simulink model "regen"  (R2025b)
settings: Solver=FixedStepAuto  StartTime=0.0  StopTime=55  FixedStep=0.005  RelTol=1e-3
InitFcn:
  | speed_min = 6;
  | bpt_fmax = 60;
  | bpt_rmax = 60;
  | voltage_max = 299;
  | pedals_max = 0;
model workspace (MAT data in the model file):
  efficiency_grid = [0  0  0  0  0  0  0  0  0  0  0; 0  0.86  0.88  0.89  0.89  0.89  0.89  0.88  0.86  0.8  0.8; 0  0.88  0.94  0.94  0.95  0.95  0.94  0.94  0.94  0.88  0.85; 0  0.88  0.94  0.95  0.96  0.96  0.96  0.96  0.95  0.94  0.86; 0  0.88  0.94  0.95  0.96  0.95  0.95  0.95  0.95  0.94  0.93; 0  0.86  0.91  0.94  0.94  0.94  0.94  0.94  0.94  0.94  0.94; 0  0.83  0.88  0.92  0.92  0.92  0.92  0.92  0.92  0.91  0.9; 0  0.8  0.86  0.86  0.86  0.86  0.86  0.86  0.86  0.86  0.86]
  rpm_grid = [0  500  1000  1500  2000  2500  3000  3500  4000  4500  5000; 0  500  1000  1500  2000  2500  3000  3500  4000  4500  5000; 0  500  1000  1500  2000  2500  3000  3500  4000  4500  5000; 0  500  1000  1500  2000  2500  3000  3500  4000  4500  5000; 0  500  1000  1500  2000  2500  3000  3500  4000  4500  5000; 0  500  1000  1500  2000  2500  3000  3500  4000  4500  5000; 0  500  1000  1500  2000  2500  3000  3500  4000  4500  5000; 0  500  1000  1500  2000  2500  3000  3500  4000  4500  5000]
  torque_grid = [0  0  0  0  0  0  0  0  0  0  0; 20  20  20  20  20  20  20  20  20  20  20; 40  40  40  40  40  40  40  40  40  40  40; 60  60  60  60  60  60  60  60  60  60  60; 80  80  80  80  80  80  80  80  80  80  80; 100  100  100  100  100  100  100  100  100  100  100; 120  120  120  120  120  120  120  120  120  120  120; 140  140  140  140  140  140  140  140  140  140  140]
undefined symbols (not defined in the file or in its folder): DiscIntNeverNeededParam
libraries: simulink x4, sdolib x2
settings Model: Creator=benjaminlevin  LastModifiedBy=benjaminlevin

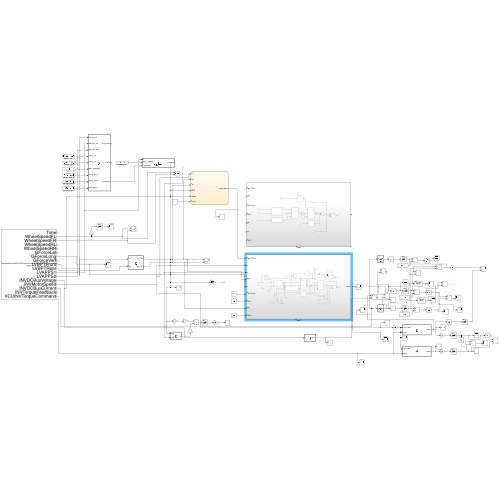
[thumbnail: Simulink's stored preview of the top-level diagram]
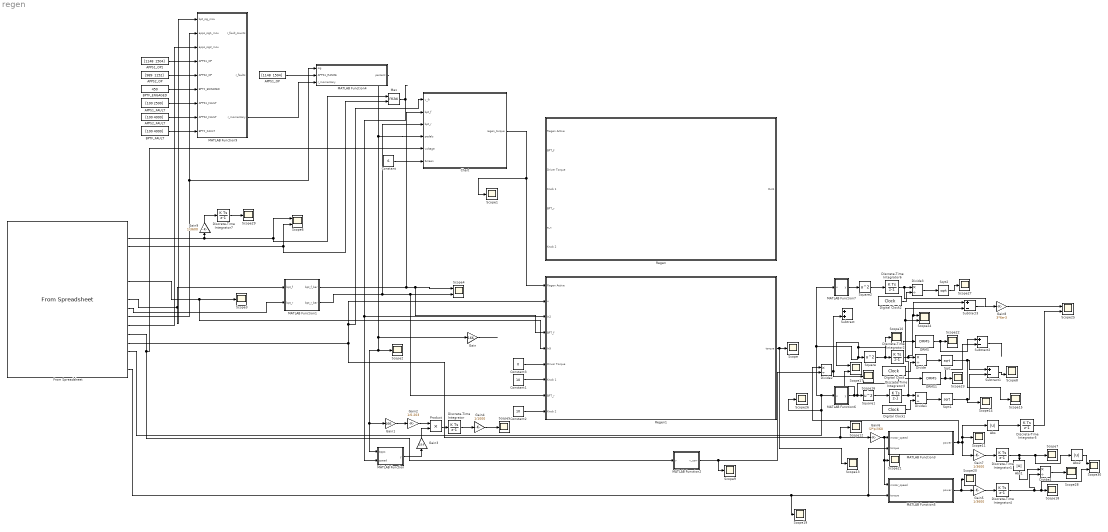
== system regen ==
  APPS1_FAULT : Constant  Value=[100 2500]  VectorParams1D=off
  APPS1_OP : Constant  Value="[1148  1504]"  VectorParams1D=off
  APPS1_OP1 : Constant  Value="[1148  1504]"  VectorParams1D=off
  APPS2_FAULT : Constant  Value=[100 4000]  VectorParams1D=off
  APPS2_OP : Constant  Value="[989  1152]"  VectorParams1D=off
  Abs : Abs  SaturateOnIntegerOverflow=off
  Abs1 : Abs  SaturateOnIntegerOverflow=off
  Abs2 : Abs  SaturateOnIntegerOverflow=off
  BPTF_ENGAGED : Constant  Value=450  VectorParams1D=off
  BPTF_FAULT : Constant  Value=[100 4000]  VectorParams1D=off
  Chart : Stateflow chart  TreatAsAtomicUnit=on
  Constant : Constant  Value=6
  Constant1 : Constant  Value=10
  Constant2 : Constant  Value=10
  Constant3 : Constant  Value=0
  DRMS : sdolib/RMS Blocks/DRMS  Ts=0.005
  DRMS1 : sdolib/RMS Blocks/DRMS  Ts=0.005
  Digital Clock : DigitalClock  SampleTime=0.005
  Digital Clock1 : DigitalClock  SampleTime=0.005
  Digital Clock2 : DigitalClock  SampleTime=0.005
  Discrete-Time Integrator{,1,4..5,7} (5 alike) : DiscreteIntegrator  SampleTime=-1  ICPrevOutput=DiscIntNeverNeededParam  ICPrevScaledInput=DiscIntNeverNeededParam
  Discrete-Time Integrator2 : DiscreteIntegrator  SampleTime=-1  SaturateOnIntegerOverflow=on  ICPrevOutput=DiscIntNeverNeededParam  ICPrevScaledInput=DiscIntNeverNeededParam
  Discrete-Time Integrator3 : DiscreteIntegrator  SampleTime=-1  SaturateOnIntegerOverflow=on  ICPrevOutput=DiscIntNeverNeededParam  ICPrevScaledInput=DiscIntNeverNeededParam
  Discrete-Time Integrator6 : DiscreteIntegrator  SampleTime=-1  SaturateOnIntegerOverflow=on  ICPrevOutput=DiscIntNeverNeededParam  ICPrevScaledInput=DiscIntNeverNeededParam
  Divide{,1..4} (5 alike) : Product  Inputs=*/
  From Spreadsheet : FromSpreadsheet  FileName=/Users/benjaminlevin/MATLAB/Projects/FormulaSAE/Simulations/regen_test2.xlsx  TreatFirstColumnAs=Data  SampleTime=0.005
  Gain : Gain  Gain=166
  Gain1 : Gain  Gain=166
  Gain2 : Gain  Gain=1/0.203
  Gain3 : Gain  Gain=1/3.6
  Gain4 : Gain  Gain=1/1000
  Gain5 : Gain  Gain=1/3600
  Gain6 : Gain  Gain=(2*pi)/60
  Gain7 : Gain  Gain=1/3600
  Gain8 : Gain  Gain=3*6e-3
  Gain9 : Gain  Gain=1/3600
  MATLAB Function : MATLAB Function  TreatAsAtomicUnit=on
  MATLAB Function1 : MATLAB Function  TreatAsAtomicUnit=on
  MATLAB Function2 : MATLAB Function  TreatAsAtomicUnit=on
  MATLAB Function3 : MATLAB Function  TreatAsAtomicUnit=on
  MATLAB Function4 : MATLAB Function  TreatAsAtomicUnit=on
  MATLAB Function5 : MATLAB Function  TreatAsAtomicUnit=on
  MATLAB Function6 : MATLAB Function  TreatAsAtomicUnit=on
  MATLAB Function7 : MATLAB Function  TreatAsAtomicUnit=on
  MATLAB Function9 : MATLAB Function  TreatAsAtomicUnit=on
  Max : MinMax  Function=max  Inputs=2
  Product : Product
  Regen : Subsystem
  Regen1 : Subsystem
  Scope{,1..3,5,7,9..16,18..23,26..29} (24 alike) : Scope
      Scope settings: ActiveDisplayYMinimum=-21.15145094913067  ActiveDisplayYMaximum=2.3501612165700738
      Scope1 settings: ActiveDisplayYMinimum=-0.12499999999999997  ActiveDisplayYMaximum=1.125
      Scope10 settings: ActiveDisplayYMinimum=-1  ActiveDisplayYMaximum=1  DataLoggingVariableName=ScopeData16
      Scope11 settings: ActiveDisplayYMinimum=-9272.4847143408551  ActiveDisplayYMaximum=1030.2760793712059  DataLoggingVariableName=ScopeData17
      Scope12 settings: ActiveDisplayYMinimum=-1  ActiveDisplayYMaximum=1  DataLoggingVariableName=ScopeData18
      Scope13 settings: ActiveDisplayYMinimum=-1  ActiveDisplayYMaximum=1  DataLoggingVariableName=ScopeData19
      Scope14 settings: ActiveDisplayYMinimum=-1  ActiveDisplayYMaximum=1  DataLoggingVariableName=ScopeData20
      Scope15 settings: ActiveDisplayYMinimum=-6.708659854939345  ActiveDisplayYMaximum=60.377938694454123  DataLoggingVariableName=ScopeData21
      Scope16 settings: ActiveDisplayYMinimum=-1  ActiveDisplayYMaximum=1  DataLoggingVariableName=ScopeData22
      Scope18 settings: ActiveDisplayYMinimum=-7.349479921094539  ActiveDisplayYMaximum=66.14531928985086  DataLoggingVariableName=ScopeData24
      Scope19 settings: ActiveDisplayYMinimum=-93.25  ActiveDisplayYMaximum=149.25  DataLoggingVariableName=ScopeData25
      Scope2 settings: ActiveDisplayYMinimum=-0.12499999999999997  ActiveDisplayYMaximum=1.125  DataLoggingVariableName=ScopeData3
      Scope20 settings: ActiveDisplayYMinimum=-2830.8048074376215  ActiveDisplayYMaximum=25477.243266938596  DataLoggingVariableName=ScopeData26
      Scope21 settings: ActiveDisplayYMinimum=-1  ActiveDisplayYMaximum=1  DataLoggingVariableName=ScopeData27
      Scope22 settings: ActiveDisplayYMinimum=-6.70865985493934  ActiveDisplayYMaximum=60.377938694454073  DataLoggingVariableName=ScopeData28
      Scope23 settings: ActiveDisplayYMinimum=-6.6179312460260808  ActiveDisplayYMaximum=59.561381214234743  DataLoggingVariableName=ScopeData29
      Scope26 settings: ActiveDisplayYMinimum=-1  ActiveDisplayYMaximum=1  DataLoggingVariableName=ScopeData32
      Scope27 settings: ActiveDisplayYMinimum=-1.016637699694753  ActiveDisplayYMaximum=9.14973929725278  DataLoggingVariableName=ScopeData33
      Scope28 settings: ActiveDisplayYMinimum=-0.011828803968027645  ActiveDisplayYMaximum=0.10645923571224883  DataLoggingVariableName=ScopeData34
      Scope29 settings: ActiveDisplayYMinimum=0.415904174307646  ActiveDisplayYMaximum=0.51853213869138126  DataLoggingVariableName=ScopeData35
      Scope3 settings: ActiveDisplayYMinimum=-1  ActiveDisplayYMaximum=1  DataLoggingVariableName=ScopeData4
      Scope5 settings: ActiveDisplayYMinimum=-43.210764305632928  ActiveDisplayYMaximum=388.89687875069643  DataLoggingVariableName=ScopeData9
      Scope7 settings: ActiveDisplayYMinimum=-5.8508187823194051  ActiveDisplayYMaximum=0.65009097581326714  DataLoggingVariableName=ScopeData13
      Scope9 settings: ActiveDisplayYMinimum=-32.999999999999993  ActiveDisplayYMaximum=307  DataLoggingVariableName=ScopeData15
  Scope{4,6,8,17,24..25,30} (7 alike) : Scope  NumInputPorts=2
      Scope17 settings: ActiveDisplayYMinimum=-2.2007545776515816  ActiveDisplayYMaximum=3.9988785651090524  DataLoggingVariableName=ScopeData23
      Scope24 settings: ActiveDisplayYMinimum=-15091.611533634048  ActiveDisplayYMaximum=135824.50380270646  DataLoggingVariableName=ScopeData30
      Scope25 settings: ActiveDisplayYMinimum=-2340.3275129277604  ActiveDisplayYMaximum=21062.947616349848  DataLoggingVariableName=ScopeData31
      Scope30 settings: ActiveDisplayYMinimum=-7.349479921094539  ActiveDisplayYMaximum=66.14531928985086  DataLoggingVariableName=ScopeData36
      Scope4 settings: ActiveDisplayYMinimum=-19.813186813186814  ActiveDisplayYMaximum=52.512820512820511  DataLoggingVariableName=ScopeData5
      Scope6 settings: ActiveDisplayYMinimum=39.9848363195723  ActiveDisplayYMaximum=55.121696594158571  DataLoggingVariableName=ScopeData12
      Scope8 settings: ActiveDisplayYMinimum=-0.082085964543487031  ActiveDisplayYMaximum=0.7387736808913834  DataLoggingVariableName=ScopeData14
  Sqrt : Sqrt
  Sqrt1 : Sqrt
  Sqrt2 : Sqrt
  Square : Math  Operator=square
  Square1 : Math  Operator=square
  Square2 : Math  Operator=square
  Subtract : Sum
  Subtract1 : Sum  Inputs=+-
  Subtract2 : Sum  Inputs=+-
  Subtract3 : Sum  Inputs=+-
  wires:
  Chart/1(regen_torque) -> Scope1/1, Regen1/1(Regen Active)
  MATLAB Function9/3(r_momentary) -> MATLAB Function4/3(r_momentary)
  APPS1_OP/1 -> MATLAB Function4/2(APPS1_RANGE)
  APPS1_OP1/1 -> MATLAB Function9/4(APPS1_OP)
  APPS2_OP/1 -> MATLAB Function9/5(APPS2_OP)
  BPTF_ENGAGED/1 -> MATLAB Function9/6(BPTF_ENGAGED)
  APPS1_FAULT/1 -> MATLAB Function9/7(APPS1_FAULT)
  APPS2_FAULT/1 -> MATLAB Function9/8(APPS2_FAULT)
  BPTF_FAULT/1 -> MATLAB Function9/9(BPTF_FAULT)
  Constant/1 -> Chart/6(Screen)
  Max/1 -> MATLAB Function/2(speed), Regen1/3(In2)
  MATLAB Function4/1(percent) -> Gain1/1, MATLAB Function/1(apps), Scope2/1, Gain/1, Chart/4(pedals)
  Gain/1 -> ?
  Constant1/1 -> Regen1/7(Knob 1)
  Constant2/1 -> Regen1/9(Knob 2)
  From Spreadsheet/2 -> Scope6/1, Max/1, Gain9/1
  From Spreadsheet/3 -> Max/2, Scope6/2
  From Spreadsheet/9 -> MATLAB Function9/1(bpt_sig_mcu), MATLAB Function1/1(bpt_f)
  From Spreadsheet/10 -> MATLAB Function1/2(bpt_r)
  From Spreadsheet/11 -> MATLAB Function4/1(sig), MATLAB Function9/2(apps_sig1_mcu)
  From Spreadsheet/12 -> MATLAB Function9/3(apps_sig2_mcu)
  From Spreadsheet/7 -> Regen1/5(In5), Scope3/1
  Constant3/1 -> Regen1/6(Driver Torque)
  MATLAB Function/1(y) -> Gain3/1
  Gain1/1 -> Gain2/1
  Product/1 -> Discrete-Time Integrator/1
  Discrete-Time Integrator/1 -> Gain4/1
  Gain2/1 -> Product/1
  Gain3/1 -> Product/2
  Gain4/1 -> Scope5/1
  MATLAB Function1/2(bpt_r_bar) -> Regen1/8(BPT_r), Scope4/2, Chart/3(bpt_r)
  MATLAB Function1/1(bpt_f_bar) -> Regen1/4(BPT_f), Scope4/1, Chart/2(bpt_f)
  Discrete-Time Integrator2/1 -> Subtract3/1, Scope24/1, Divide/1
  From Spreadsheet/14 -> Scope12/1, Gain6/1, Regen1/2(u), Chart/1(v_fr)
  MATLAB Function3/1(power) -> Divide2/1, Abs/1, Scope11/1, Gain7/1
  Regen1/1(torque) -> Scope13/1, Scope/1
  Divide/1 -> Sqrt/1
  Square/1 -> Discrete-Time Integrator2/1, Scope10/1
  Digital Clock1/1 -> Divide1/2
  Square1/1 -> Discrete-Time Integrator3/1
  Divide1/1 -> Sqrt1/1
  Digital Clock/1 -> Divide/2
  From Spreadsheet/15 -> Scope26/1, MATLAB Function7/1(u), Scope17/1, DRMS/1, Square/1, MATLAB Function6/1(u)
  From Spreadsheet/13 -> MATLAB Function2/1(v), Chart/5(voltage)
  Divide2/1 -> Subtract/2, Scope16/1
  Sqrt1/1 -> Scope14/1, Subtract1/2
  Sqrt/1 -> Scope15/1, Subtract1/1
  Subtract1/1 -> Scope8/2
  MATLAB Function2/1(v_corr) -> Scope9/1, Divide2/2
  Discrete-Time Integrator3/1 -> Scope24/2, Subtract3/2, Divide1/1
  Gain6/1 -> Scope21/1, MATLAB Function5/1(motor_speed), MATLAB Function3/1(motor_speed)
  Gain7/1 -> Discrete-Time Integrator1/1
  Gain5/1 -> Discrete-Time Integrator4/1
  Discrete-Time Integrator4/1 -> Divide4/2, Scope30/2, Scope18/1
  From Spreadsheet/17 -> Scope19/1, MATLAB Function3/2(torque), MATLAB Function5/2(torque)
  MATLAB Function5/1(power) -> Scope20/1, Gain5/1
  DRMS1/1 -> Subtract2/2, Scope23/1
  DRMS/1 -> Subtract2/1, Scope22/1
  Subtract2/1 -> ?
  Subtract3/1 -> ?
  Gain8/1 -> Scope25/1
  Discrete-Time Integrator5/1 -> Scope25/2
  Abs/1 -> Discrete-Time Integrator5/1
  MATLAB Function6/1(y) -> Scope17/2, DRMS1/1, Square1/1
  Digital Clock2/1 -> Divide3/2
  Divide3/1 -> Sqrt2/1
  Discrete-Time Integrator6/1 -> Gain8/1, Divide3/1
  Square2/1 -> Discrete-Time Integrator6/1
  MATLAB Function7/1(y) -> Square2/1
  Sqrt2/1 -> Scope27/1
  Abs1/1 -> Divide4/1
  Divide4/1 -> Scope28/1
  Discrete-Time Integrator7/1 -> Scope29/1
  Gain9/1 -> Discrete-Time Integrator7/1
  Discrete-Time Integrator1/1 -> Abs1/1, Abs2/1, Scope7/1
  Abs2/1 -> Scope30/1

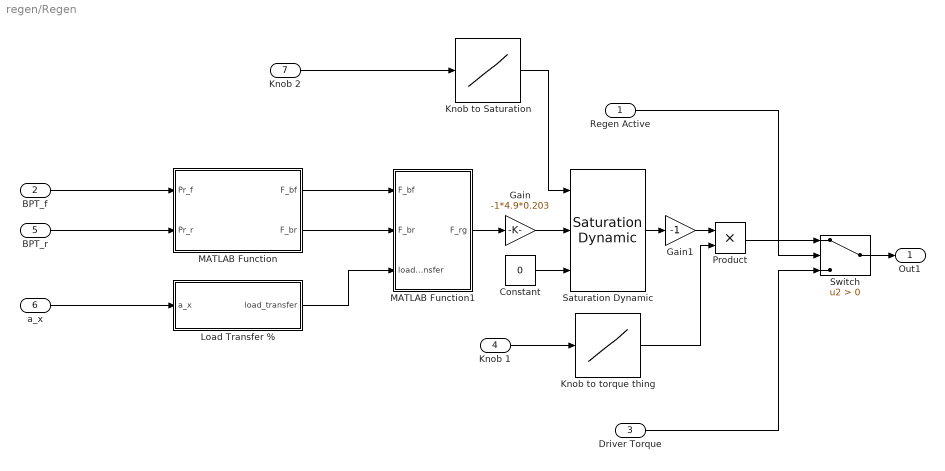
== system regen/Regen ==
  Regen Active : Inport
  BPT_f : Inport  Port=2
  Driver Torque : Inport  Port=3
  Knob 1 : Inport  Port=4
  BPT_r : Inport  Port=5
  a_x : Inport  Port=6
  Knob 2 : Inport  Port=7
  Constant : Constant  Value=0
  Gain : Gain  Gain=-1*4.9*0.203
  Gain1 : Gain  Gain=-1
  Knob to Saturation : Lookup_n-D  NumberOfTableDimensions=1  BreakpointsForDimension1=[1 10]  Table=[16.6 83]  InternalRulePriority=Speed  RndMeth=Simplest
  Knob to torque thing : Lookup_n-D  NumberOfTableDimensions=1  BreakpointsForDimension1=[1 10]  Table=[0 3]  InternalRulePriority=Speed  RndMeth=Simplest
  Load Transfer % : MATLAB Function  TreatAsAtomicUnit=on
  MATLAB Function : MATLAB Function  TreatAsAtomicUnit=on
  MATLAB Function1 : MATLAB Function  TreatAsAtomicUnit=on
  Product : Product
  Saturation Dynamic : simulink/Discontinuities/Saturation Dynamic  OutMin=[]  OutMax=[]  OutDataTypeStr=Inherit: Same as second input  OutDataType=fixdt(1, 16)  OutScaling=2^-10  DoSatur=off
  Switch : Switch  Criteria=u2 > Threshold  SaturateOnIntegerOverflow=off  InputSameDT=off
  Out1 : Outport
  wires:
  Switch/1 -> Out1/1
  Driver Torque/1 -> Switch/3
  Saturation Dynamic/1 -> Gain1/1
  Regen Active/1 -> Switch/2
  Knob to torque thing/1 -> Product/2
  Knob 1/1 -> Knob to torque thing/1
  BPT_f/1 -> MATLAB Function/1(Pr_f)
  BPT_r/1 -> MATLAB Function/2(Pr_r)
  a_x/1 -> Load Transfer %/1(a_x)
  MATLAB Function/1(F_bf) -> MATLAB Function1/1(F_bf)
  MATLAB Function/2(F_br) -> MATLAB Function1/2(F_br)
  Load Transfer %/1(load_transfer) -> MATLAB Function1/3(load_transfer)
  MATLAB Function1/1(F_rg) -> Gain/1
  Gain/1 -> Saturation Dynamic/2
  Gain1/1 -> Product/1
  Constant/1 -> Saturation Dynamic/3
  Knob 2/1 -> Knob to Saturation/1
  Knob to Saturation/1 -> Saturation Dynamic/1
  Product/1 -> Switch/1

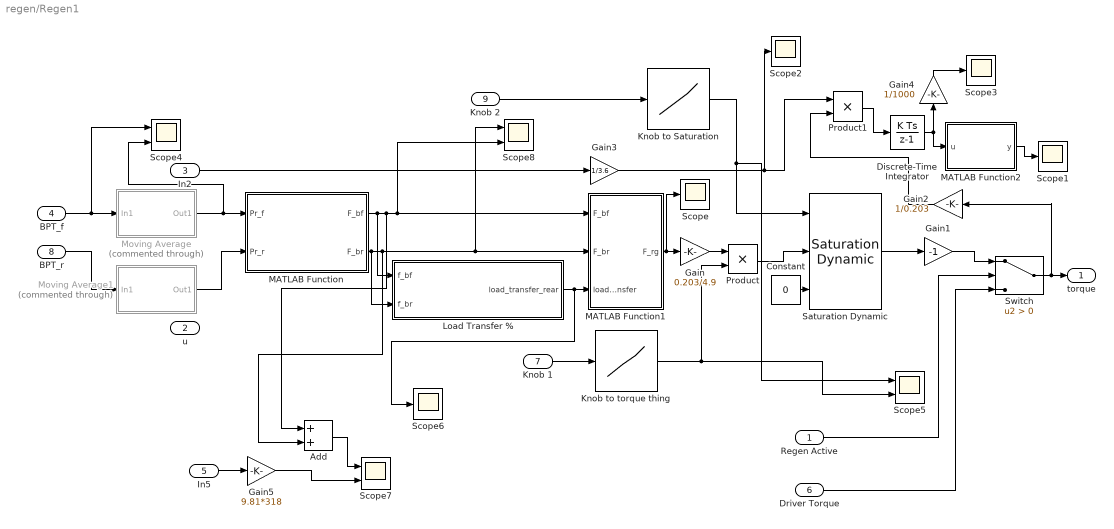
== system regen/Regen1 ==
  Regen Active : Inport
  u : Inport  Port=2
  In2 : Inport  Port=3
  BPT_f : Inport  Port=4
  In5 : Inport  Port=5
  Driver Torque : Inport  Port=6
  Knob 1 : Inport  Port=7
  BPT_r : Inport  Port=8
  Knob 2 : Inport  Port=9
  Add : Sum
  Constant : Constant  Value=0
  Discrete-Time Integrator : DiscreteIntegrator  SampleTime=-1  ICPrevOutput=DiscIntNeverNeededParam  ICPrevScaledInput=DiscIntNeverNeededParam
  Gain : Gain  Gain=0.203/4.9
  Gain1 : Gain  Gain=-1
  Gain2 : Gain  Gain=1/0.203
  Gain3 : Gain  Gain=1/3.6
  Gain4 : Gain  Gain=1/1000
  Gain5 : Gain  Gain=9.81*318
  Knob to Saturation : Lookup_n-D  NumberOfTableDimensions=1  BreakpointsForDimension1=[1 10]  Table=[16.6 83]  InternalRulePriority=Speed  RndMeth=Simplest
  Knob to torque thing : Lookup_n-D  NumberOfTableDimensions=1  BreakpointsForDimension1=[1 10]  Table=[0 3]  InternalRulePriority=Speed  RndMeth=Simplest
  Load Transfer % : MATLAB Function  TreatAsAtomicUnit=on
  MATLAB Function : MATLAB Function  TreatAsAtomicUnit=on
  MATLAB Function1 : MATLAB Function  TreatAsAtomicUnit=on
  MATLAB Function2 : MATLAB Function  TreatAsAtomicUnit=on
  Moving Average : Subsystem  Commented=through
  Moving Average1 : Subsystem  Commented=through
  Product : Product
  Product1 : Product
  Saturation Dynamic : simulink/Discontinuities/Saturation Dynamic  OutMin=[]  OutMax=[]  OutDataTypeStr=Inherit: Same as second input  OutDataType=fixdt(1, 16)  OutScaling=2^-10  DoSatur=off
  Scope{,1..3,6} (5 alike) : Scope
      Scope settings: ActiveDisplayYMinimum=-590.48960894112406  ActiveDisplayYMaximum=472.92488421823089  DataLoggingVariableName=ScopeData2
      Scope1 settings: ActiveDisplayYMinimum=-1  ActiveDisplayYMaximum=1  DataLoggingVariableName=ScopeData6
      Scope2 settings: DataLoggingVariableName=ScopeData7
      Scope3 settings: ActiveDisplayYMinimum=-0.93739008484543129  ActiveDisplayYMaximum=-0.38106337616278252  DataLoggingVariableName=ScopeData8
      Scope6 settings: ActiveDisplayYMinimum=0.41919170740939254  ActiveDisplayYMaximum=0.47317190084232807  DataLoggingVariableName=ScopeData37
  Scope{4..5,7..8} (4 alike) : Scope  NumInputPorts=2
      Scope4 settings: ActiveDisplayYMinimum=-97.374999999999972  ActiveDisplayYMaximum=866.375  DataLoggingVariableName=ScopeData10
      Scope5 settings: DataLoggingVariableName=ScopeData11
      Scope7 settings: ActiveDisplayYMinimum=-4051.4963955380586  ActiveDisplayYMaximum=2772.0035598425193  DataLoggingVariableName=ScopeData38
      Scope8 settings: ActiveDisplayYMinimum=87.082901447640324  ActiveDisplayYMaximum=1865.6198504440433  DataLoggingVariableName=ScopeData39
  Switch : Switch  Criteria=u2 > Threshold  SaturateOnIntegerOverflow=off  InputSameDT=off
  torque : Outport
  wires:
  Switch/1 -> Gain2/1, torque/1
  Driver Torque/1 -> Switch/3
  Saturation Dynamic/1 -> Gain1/1
  Regen Active/1 -> Switch/2
  Knob to torque thing/1 -> Product/2, Scope5/2
  Knob 1/1 -> Knob to torque thing/1
  BPT_f/1 -> Scope4/1, Moving Average/1(In1)
  BPT_r/1 -> Moving Average1/1(In1)
  MATLAB Function/1(F_bf) -> Add/1, Scope8/2, MATLAB Function1/1(F_bf), Load Transfer %/1(f_bf)
  MATLAB Function/2(F_br) -> Add/2, Scope8/1, MATLAB Function1/2(F_br), Load Transfer %/2(f_br)
  Gain/1 -> Product/1
  Constant/1 -> Saturation Dynamic/3
  Knob 2/1 -> Knob to Saturation/1
  Knob to Saturation/1 -> Scope5/1, Saturation Dynamic/1
  Gain1/1 -> Switch/1
  MATLAB Function1/1(F_rg) -> Gain/1, Scope/1
  Discrete-Time Integrator/1 -> Gain4/1, MATLAB Function2/1(u)
  MATLAB Function2/1(y) -> Scope1/1
  In2/1 -> Gain3/1
  Product1/1 -> Discrete-Time Integrator/1
  Gain2/1 -> Product1/2
  Gain3/1 -> Scope2/1, Product1/1
  Gain4/1 -> Scope3/1
  Moving Average/1(Out1) -> Scope4/2, MATLAB Function/1(Pr_f)
  Moving Average1/1(Out1) -> MATLAB Function/2(Pr_r)
  Product/1 -> Saturation Dynamic/2
  Load Transfer %/1(load_transfer_rear) -> Scope6/1, MATLAB Function1/3(load_transfer)
  In5/1 -> Gain5/1
  Add/1 -> Scope7/1
  Gain5/1 -> Scope7/2

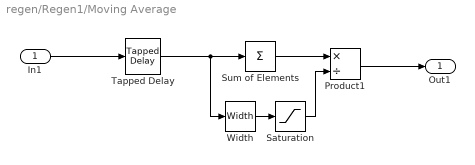
== system regen/Regen1/Moving Average ==
  In1 : Inport
  Product1 : Product  Inputs=*/
  Saturation : Saturate  UpperLimit=inf  LowerLimit=1
  Sum of Elements : Sum  Inputs=+
  Tapped Delay : simulink/Discrete/Tapped Delay  vinit=0.0  samptime=-1  NumDelays=10  DelayOrder=Oldest  includeCurrent=on
  Width : Width
  Out1 : Outport
  wires:
  Tapped Delay/1 -> Width/1, Sum of Elements/1
  Sum of Elements/1 -> Product1/1
  Product1/1 -> Out1/1
  In1/1 -> Tapped Delay/1
  Width/1 -> Saturation/1
  Saturation/1 -> Product1/2

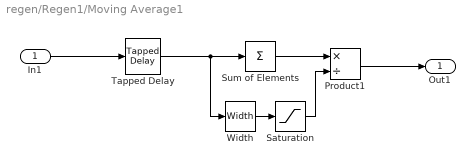
== system regen/Regen1/Moving Average1 ==
  In1 : Inport
  Product1 : Product  Inputs=*/
  Saturation : Saturate  UpperLimit=inf  LowerLimit=1
  Sum of Elements : Sum  Inputs=+
  Tapped Delay : simulink/Discrete/Tapped Delay  vinit=0.0  samptime=-1  NumDelays=10  DelayOrder=Oldest  includeCurrent=on
  Width : Width
  Out1 : Outport
  wires:
  Tapped Delay/1 -> Width/1, Sum of Elements/1
  Sum of Elements/1 -> Product1/1
  Product1/1 -> Out1/1
  In1/1 -> Tapped Delay/1
  Width/1 -> Saturation/1
  Saturation/1 -> Product1/2

== matlab function regen/Regen1/Load Transfer % ==
  data: f_bf input; load_transfer_rear output; f_br input
function load_transfer_rear = fcn(f_bf, f_br)
m = 250+68; %Mass with driver weight
a = 1.530/2; %Distance cg to front axle with load distribution of 0.5
h = 0.249; %Height of CG
l = 1.530; %Length of wheelbase
total_f = f_bf + f_br;
g = 9.81;
load_transfer_rear = abs((a*m*g)/l-(total_f*h)/l)/(m*g);

== matlab function regen/Regen1/MATLAB Function ==
  data: F_bf output; Pr_f input; F_br output; Pr_r input
function [F_bf,F_br] = fcn(Pr_f,Pr_r)
mu = 0.410;
r_rotor = 76.96e-3; %m, effective rotor radius
r_tire = 203.2e-3; %m
A_r = 1816e-6; %m^2
%psi_to_bar = 1/14.503;
%maybe ((1/BB_e)-1), MIT paper, now is just some variable 0 to 1 minus 1
F_br = (2*mu*(r_rotor/r_tire)*A_r*Pr_r)*(100000);
F_bf = (2*mu*(r_rotor/r_tire)*A_r*Pr_f)*(100000);

== matlab function regen/Regen1/MATLAB Function1 ==
  data: F_rg output; F_bf input; F_br input; load_transfer input
function F_rg = fcn(F_bf,F_br,load_transfer)
F_rg = (F_bf+F_br)*load_transfer-F_br;

== matlab function regen/MATLAB Function4 ==
  data: sig input; APPS1_RANGE input; r_momentary input; percent output
function percent = map_apps1(sig, APPS1_RANGE, r_momentary)

DZ_BOT = .05; %rosnel changed to .05 was .1 
DZ_TOP = .05; 

APPS_BOTTOM = APPS1_RANGE(1) + DZ_BOT * (APPS1_RANGE(2) - APPS1_RANGE(1)) ;
APPS_TOP    = APPS1_RANGE(2) - DZ_TOP * (APPS1_RANGE(2) - APPS1_RANGE(1)) ;

if (sig < APPS_BOTTOM) || r_momentary(1) || r_momentary(2)
    percent = 0;
elseif sig > APPS_TOP
    percent = 1;
else
    percent = (double(sig) - APPS_BOTTOM) / (APPS_TOP - APPS_BOTTOM);
end

== matlab function regen/Regen1/MATLAB Function2 ==
  settings: updateMethod=DISCRETE
  data: u input; y output
function y = fcn(u)
persistent e;
if isempty(e)
    e = 0;
end
e = e + u;
y = e/1000;

== matlab function regen/MATLAB Function ==
  data: apps input; y output; speed input
function y = fcn(apps,speed)
if apps > 0
y = speed;
else
 y = 0;
end

== matlab function regen/MATLAB Function9 ==
  data: r_fault_counts output; r_faults output; bpt_sig_mcu input; apps_sig1_mcu input; apps_sig2_mcu input; APPS1_OP input; APPS2_OP input; BPTF_ENGAGED input; APPS1_FAULT input; APPS2_FAULT input; BPTF_FAULT input; r_momentary output
function [r_fault_counts, r_faults, r_momentary] = fcn(bpt_sig_mcu, apps_sig1_mcu, apps_sig2_mcu, APPS1_OP, APPS2_OP, BPTF_ENGAGED, APPS1_FAULT, APPS2_FAULT, BPTF_FAULT)
%#codegen
%To map voltages / integers:
%Pre step down voltages (from sensors, range 0 to 5 V) * 2/3 -> Post step down voltages (0 to 3.3 V, used by mcu)
%Post step down voltages * (4096 / 3.3) -> uint16 (integer) value of variables
%Note: Some values are tweaked after testing to handle noise. 455 -> 435, 0.1 -> 0.13, etc. All values can and should be optimized from testing, especially from testing on the car

%Current operating range (MCU): 0.32 V to 2.67 V
%Brakes considered pressed: 0.40 V
%typical MCU noise: +- 0.03V

persistent fault_counts;
persistent faults;

FAULT_LIMITS = [10, 10, 10, 10, 10, 10, 10, 1];

% initialize persistents
if isempty(fault_counts)
    fault_counts = zeros(1,8);
end

if isempty(faults)
    faults = [false, false, false, false, false, false, false, false];
end

apps1_percent_pressed = (double(apps_sig1_mcu) - APPS1_OP(1))/(APPS1_OP(2) - APPS1_OP(1)); % current travel divided by range of travel
apps2_percent_pressed = (double(apps_sig2_mcu) - APPS2_OP(1))/(APPS2_OP(2) - APPS2_OP(1));

% Clear fault case 8 (two pedals) when apps goes below 5% travel
if (apps1_percent_pressed < 0.05)
    faults(8) = 0;
    fault_counts(8) = 0;
end

% Cases 1-6: APPS or BPT out of operating range (sensor failure)
out_of_bounds = [apps_sig1_mcu < APPS1_FAULT(1), apps_sig1_mcu > APPS1_FAULT(2), ...
                 apps_sig2_mcu < APPS2_FAULT(1), apps_sig2_mcu > APPS2_FAULT(2), ...
                 bpt_sig_mcu   < BPTF_FAULT(1),  bpt_sig_mcu   > BPTF_FAULT(2)];
% Case 7: Both APPS sensors differ by more than 10% for more than 100ms. 
apps_disagree = abs(apps1_percent_pressed - apps2_percent_pressed) > 0.1;
% Case 8: If APPS is more than 25% pressed and brakes are pressed.
two_pedal = (apps1_percent_pressed >= 0.25) && (bpt_sig_mcu >= BPTF_ENGAGED);

conditions = [out_of_bounds, apps_disagree, two_pedal];

r_momentary = conditions;

conditions(8) = conditions(8) || faults(8); % Case 8 is sticky

% if condition is met but haven't yet triggered fault, increment fault_count.
% if condition is met but already in fault, leave fault_count the same (to
% prevent overflow)
% if condition is not met, zero the count
fault_counts = conditions .* (fault_counts + not(faults));
faults = fault_counts >= FAULT_LIMITS;

r_fault_counts = fault_counts;
r_faults = faults;

== matlab function regen/MATLAB Function3 ==
  data: motor_speed input; power output; torque input; efficiency_grid parameter; torque_grid parameter; rpm_grid parameter
function power = fcn(motor_speed,torque,efficiency_grid, torque_grid, rpm_grid)
if torque < 0
    eff = interp2(rpm_grid,torque_grid,efficiency_grid,motor_speed,-torque,'linear');
else
    eff=0;
end
if isnan(eff)
    eff = 0;
end
power = motor_speed*torque*eff; %rpm * Nm * eff

== matlab function regen/MATLAB Function2 ==
  data: v input; v_corr output
function v_corr = fcn(v)
if v == 0
    v_corr = 273; %Volts
else
    v_corr = v;
end

== matlab function regen/MATLAB Function5 ==
  data: motor_speed input; power output; torque input; efficiency_grid parameter; torque_grid parameter; rpm_grid parameter
function power = fcn(motor_speed,torque,efficiency_grid, torque_grid, rpm_grid)
if torque > 0
    eff = interp2(rpm_grid,torque_grid,efficiency_grid,motor_speed,torque,'linear');
else
    eff = 0;
end
if isnan(eff)
    eff = 0;
end
power = motor_speed*torque*eff; %rpm * Nm * eff

== matlab function regen/MATLAB Function6 ==
  data: u input; y output
function y = fcn(u)
if u > 0
    y = u;
else
    y = 0;
end

== matlab function regen/MATLAB Function7 ==
  data: u input; y output
function y = fcn(u)
if u < 0
    y = u;
else
    y = 0;
end

== matlab function regen/MATLAB Function1 ==
  data: bpt_f input; bpt_f_bar output; bpt_r input; bpt_r_bar output
function [bpt_f_bar,bpt_r_bar] = fcn(bpt_f,bpt_r)
bpt_f_bar = (((bpt_f/4095)*3.3*4)-0.5)*25;
bpt_r_bar = (((bpt_r/4095)*3.3*4)-0.5)*25;

== matlab function regen/Regen/Load Transfer % ==
  data: a_x input; load_transfer output
function load_transfer = fcn(a_x)
m = 250+68; %Mass with driver weight
a = 1.530/2; %Distance cg to front axle with load distribution of 0.5
h = 0.249; %Height of CG
l = 1.530; %Length of wheelbase
load_transfer = abs(a_x*h/l);

== matlab function regen/Regen/MATLAB Function ==
  data: F_bf output; Pr_f input; F_br output; Pr_r input
function [F_bf,F_br] = fcn(Pr_f,Pr_r)
mu = 0.410;
r_rotor = 76.96; %mm, effective rotor radius
A_r = 1816; %mm^2
psi_to_bar = 1/14.503;
%maybe ((1/BB_e)-1), MIT paper, now is just some variable 0 to 1 minus 1
F_br = (2*mu*r_rotor*A_r*Pr_r*psi_to_bar)/(10000);
F_bf = (2*mu*r_rotor*A_r*Pr_f*psi_to_bar)/(10000);

== stateflow chart regen/Chart ==
  state REGEN_AVAILABLE
    regen_torque = 1;
  state REGEN_OFF
    regen_torque = 0;
  state REGEN_NOT_AVAILABLE
    regen_torque = 0;
  (default) -> REGEN_OFF
  REGEN_AVAILABLE -> REGEN_OFF [order 1] : [Screen <= 5]
  REGEN_NOT_AVAILABLE -> REGEN_OFF [order 1] : [Screen <= 5]
  REGEN_OFF -> REGEN_NOT_AVAILABLE : [Screen > 5]
  REGEN_NOT_AVAILABLE -> REGEN_AVAILABLE [order 2] : [v_fr > 700 & bpt_f > 5 & bpt_r > 3 & voltage <  300 & pedals <= 0]
  REGEN_AVAILABLE -> REGEN_NOT_AVAILABLE [order 2] : [v_fr <= 700 || bpt_f <= 5 || bpt_r <= 3 || voltage >= 300 || pedals > 0]
  data: v_fr input; bpt_f input; bpt_r input; pedals input; voltage input; Screen input; regen_torque output double; pedals_max parameter; voltage_max parameter double; speed_min parameter

== matlab function regen/Regen/MATLAB Function1 ==
  data: F_rg output; F_bf input; F_br input; load_transfer input
function F_rg = fcn(F_bf,F_br,load_transfer)
gain = (0.5 - load_transfer)/(0.5+load_transfer);
F_rg = F_bf*gain-F_br;
